simulink model "Phase3_Model"  (R2022b)
settings: Solver=ode4  StartTime=0.0  StopTime=40  FixedStep=Ts  RelTol=1e-3
values from neighbouring files (symbols this model uses):
  Kf = place(A, B, ps)    [params.m]
  Ph = [0.034057459922 0.0150401592064 0.0617628844395 0.00121596441585 1.86639826206 0.0157647906199]    [ph.mat]
  q20 = X0(2)    [params.m]
  X0 = x0_up_1    [params.m]
settings Model: Creator=shahin  LastModifiedBy=farjadnm
settings DataIOCC: ReturnWorkspaceOutputs=off

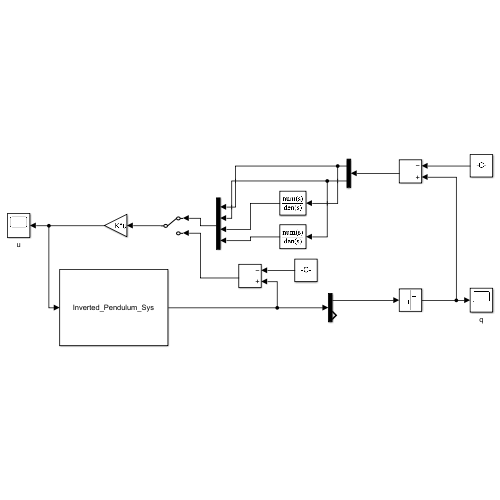
[thumbnail: Simulink's stored preview of the top-level diagram]
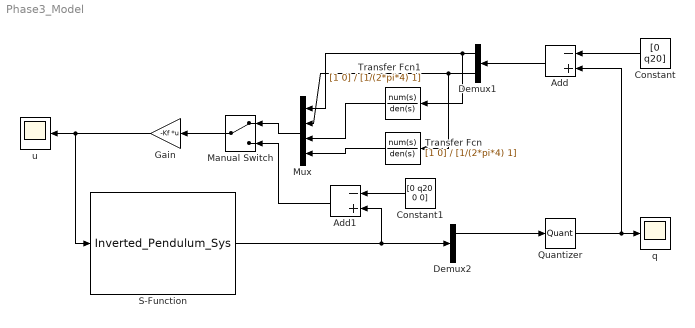
== system Phase3_Model ==
  Add : Sum  Inputs=-+
  Add1 : Sum  Inputs=-+
  Constant : Constant  Value="[0  q20]"
  Constant1 : Constant  Value="[0  q20 0 0]"
  Demux1 : Demux  Outputs=2
  Demux2 : Demux  Outputs=2
  Gain : Gain  Gain=-Kf  Multiplication=Matrix(K*u)
  Manual Switch : ManualSwitch
  Mux : Mux
  Quantizer : Quantizer  QuantizationInterval="[2*pi/2048  2*pi/2048]"
  S-Function : S-Function  FunctionName=Inverted_Pendulum_Sys  Parameters=X0,Ph  SFunctionDeploymentMode=off  EnableBusSupport=off
  Transfer Fcn : TransferFcn  Numerator=[1 0]  Denominator=[1/(2*pi*4) 1]
  Transfer Fcn1 : TransferFcn  Numerator=[1 0]  Denominator=[1/(2*pi*4) 1]
  q : Scope
  u : Scope
  wires:
  Demux2/1 -> Quantizer/1
  S-Function/1 -> Add1/2, Demux2/1
  Gain/1 -> u/1, S-Function/1
  Demux1/2 -> Mux/2, Transfer Fcn/1
  Demux1/1 -> Mux/1, Transfer Fcn1/1
  Transfer Fcn/1 -> Mux/4
  Transfer Fcn1/1 -> Mux/3
  Add/1 -> Demux1/1
  Quantizer/1 -> Add/2, q/1
  Constant/1 -> Add/1
  Constant1/1 -> Add1/1
  Manual Switch/1 -> Gain/1
  Mux/1 -> Manual Switch/1
  Add1/1 -> Manual Switch/2
